simulink model "PMSM_LPVmethods_checked"  (R2023b)
settings: Solver=ode4  StartTime=0.0  StopTime=15  FixedStep=1e-4  RelTol=1e-3
undefined symbols (not defined in the file): Ae1, Ae2, Ae3, Ae4, B, ControlMode_Elec, ControlMode_Mech, Current_Control, J, K1, k1_CST, K2, K3, K4, kd_elec, ki_elec, Km, kp_elec, L, Nr, OmegaStar_Selector, R, sigma1, sigma2, theta0, Vhatinv, Vmax
libraries: simulink x8, slpidlib x2
settings Model: Creator=ghwls  LastModifiedBy=HoLab
settings SolverCC: AlgebraicLoopSolver=TrustRegion
settings DataIOCC: SaveFormat=StructureWithTime  ReturnWorkspaceOutputs=off
settings DebuggingCC: UnconnectedInputMsg=warning  UnconnectedOutputMsg=warning  UnconnectedLineMsg=warning  ArithmeticOperatorsInVariantConditions=warning
settings ModelReferenceCC: EnableRefExpFcnMdlSchedulingChecks=on
settings SFSimCC: CustomCodeUndefinedFunction=UseInterfaceOnly

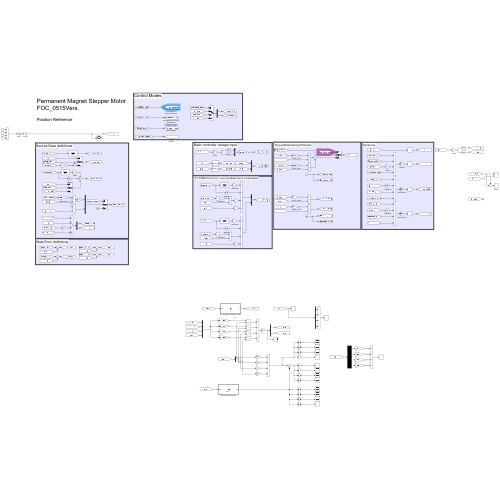
[thumbnail: Simulink's stored preview of the top-level diagram]
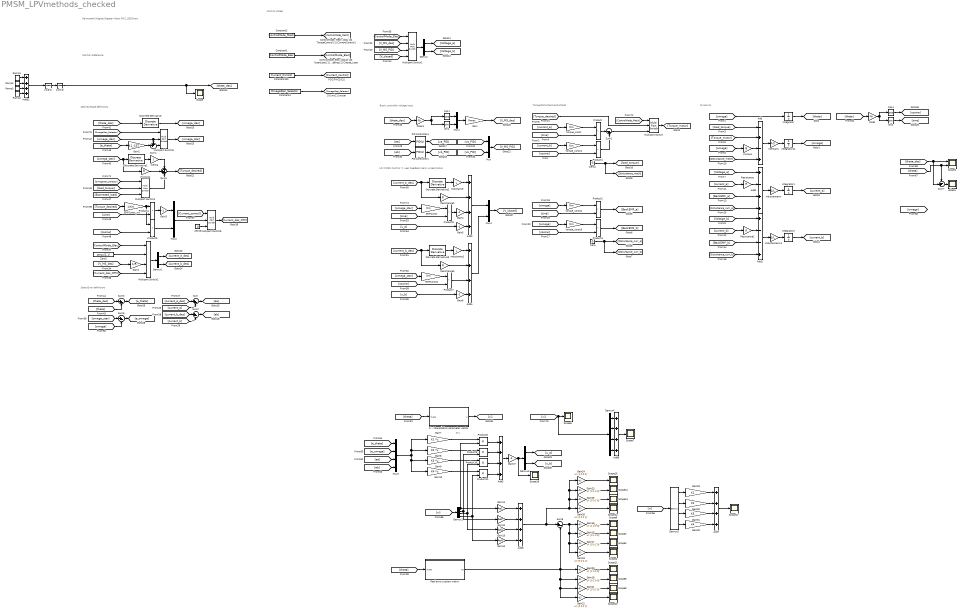
== system PMSM_LPVmethods_checked ==
  note: 2*1
  note: Control Modes
  note: Dynamics
  note: Permanent Magnet Stepper Motor
      | FOC_0515Vers.
  note: Torque/Disturbances/Purterbs
  note: Position Reference
  note: Desired State definitions
  note: Basic controller voltage input
  note: State Error definitions
  note: LPV PMSM Control (Y. Lee) Feedback Semi Liniearization
  Add : Sum  Inputs=-+-+
  Add1 : Sum  Inputs=+-++
  Add2 : Sum  Inputs=+--+
  Add3 : Sum  Inputs=++++
  Add{4..8,32} (6 alike) : Sum  Inputs=4
  Constant1 : Constant  Value=ControlMode_Elec
  Constant100 : Constant  Value=Current_Control
  Constant2 : Constant  Value=ControlMode_Mech
  Constant4 : Constant  Value=OmegaStar_Selector
  Cos1 : Trigonometry  Operator=cos
  Cos4 : Trigonometry  Operator=cos
  Demux : Demux  Outputs=2
  Demux1 : Demux  Outputs=2
  Demux2 : Demux
  Demux3 : Demux  Outputs=2
  Demux4 : Demux
  Demux5 : Demux
  Discrete Derivative{,1..3} (4 alike) : simulink/Discrete/Discrete Derivative  gainval=1.0  ICPrevScaledInput=0.0  OutMin=[]  OutMax=[]  OutDataType=fixdt(1, 16)  OutScaling=2^-10  DoSatur=off
  EMFConst : Gain  Gain=Km
  EMFConst2 : Gain  Gain=Km
  EMFConst_Inv : Gain  Gain=1/Km
  Gain : Gain  Gain=Vmax
  Gain1 : Gain  Gain=1/R
  Gain10 : Gain  Gain=K4  Multiplication=Matrix(K*u) (u vector)
  Gain11 : Gain  Gain=Ae1
  Gain12 : Gain  Gain=Ae2
  Gain13 : Gain  Gain=Ae3
  Gain14 : Gain  Gain=Ae4
  Gain15 : Gain  Gain=[0 1 0 0]'  Multiplication=Matrix(u*K)
  Gain16 : Gain  Gain=[1 0 0 0]'  Multiplication=Matrix(u*K)
  Gain17 : Gain  Gain=[0 0 1 0]'  Multiplication=Matrix(u*K)
  Gain18 : Gain  Gain=[0 0 0 1]'  Multiplication=Matrix(u*K)
  Gain19 : Gain  Gain=[0 1 0 0]'  Multiplication=Matrix(u*K)
  Gain2 : Gain  Gain=k1_CST
  Gain20 : Gain  Gain=[1 0 0 0]'  Multiplication=Matrix(u*K)
  Gain21 : Gain  Gain=[0 0 1 0]'  Multiplication=Matrix(u*K)
  Gain22 : Gain  Gain=[0 0 0 1]'  Multiplication=Matrix(u*K)
  Gain23 : Gain  Gain=[0 1 0 0]'  Multiplication=Matrix(u*K)
  Gain24 : Gain  Gain=[1 0 0 0]'  Multiplication=Matrix(u*K)
  Gain25 : Gain  Gain=[0 0 1 0]'  Multiplication=Matrix(u*K)
  Gain26 : Gain  Gain=[0 0 0 1]'  Multiplication=Matrix(u*K)
  Gain{3..6,27} (5 alike) : Gain  Gain=-1
  Gain28 : Gain  Gain=K4
  Gain29 : Gain  Gain=K1
  Gain30 : Gain  Gain=K2
  Gain31 : Gain  Gain=K3
  Gain7 : Gain  Gain=K1  Multiplication=Matrix(K*u) (u vector)
  Gain8 : Gain  Gain=K2  Multiplication=Matrix(K*u) (u vector)
  Gain9 : Gain  Gain=K3  Multiplication=Matrix(K*u) (u vector)
  Inductance : Gain  Gain=L
  Inductance1 : Gain  Gain=L
  InductanceInv : Gain  Gain=1/L
  InductanceInv1 : Gain  Gain=1/L
  Inertia : Gain  Gain=J
  InertiaInv : Gain  Gain=1/J
  Integrator : Integrator  InitialCondition=theta0
  Integrator1 : Integrator
  Integrator11 : Integrator
  Integrator2 : Integrator
  Multiport Switch{,3..5} (4 alike) : MultiPortSwitch  DataPortOrder=Zero-based contiguous  Inputs=2  zeroidx=on  SaturateOnIntegerOverflow=off  InputSameDT=off
  Multiport Switch1 : MultiPortSwitch  DataPortOrder=Zero-based contiguous  zeroidx=on  SaturateOnIntegerOverflow=off  InputSameDT=off
  Multiport Switch2 : MultiPortSwitch  DataPortOrder=Zero-based contiguous  zeroidx=on  SaturateOnIntegerOverflow=off  InputSameDT=off
  Mux{,1..2,4} (4 alike) : Mux  Inputs=2
  Mux3 : Mux
  PID Controller1 : slpidlib/PID Controller  Controller=PID  Form=Parallel  TimeDomain=Continuous-time  UseExternalTs=off  SampleTime=-1  IntegratorMethod=Forward Euler  FilterMethod=Forward Euler  ControllerParametersSource=internal  P=kp_elec  I=ki_elec  UseKiTs=off  D=kd_elec  N=100  UseFilter=on  TunerSelectOption=Transfer Function Based (PID Tuner App)  ZeroCross=off  InitialConditionSource=internal  InitialConditionForIntegrator=0  InitialConditionForFilter=0  DifferentiatorICPrevScaledInput=0  ExternalReset=none  TrackingMode=off  Kt=1  LimitOutput=off  SatLimitsSource=internal  UpperSaturationLimit=inf  LowerSaturationLimit=-inf  LinearizeAsGain=on  AntiWindupMode=none  Kb=1  LimitIntegrator=off  UpperIntegratorSaturationLimit=inf  LowerIntegratorSaturationLimit=-inf  POutMin=[]  POutMax=[]  IOutMin=[]  IOutMax=[]  DOutMin=[]  DOutMax=[]  NOutMin=[]  NOutMax=[]  SumOutMin=[]  SumOutMax=[]  SaturationOutMin=[]  SaturationOutMax=[]  PParamMin=[]  PParamMax=[]  IParamMin=[]  IParamMax=[]  DParamMin=[]  DParamMax=[]  NParamMin=[]  NParamMax=[]  KbParamMin=[]  KbParamMax=[]  KtParamMin=[]  KtParamMax=[]  KbOutMin=[]  KbOutMax=[]  KtOutMin=[]  KtOutMax=[]  IntegratorOutMin=[]  IntegratorOutMax=[]  FilterOutMin=[]  FilterOutMax=[]  SumI1OutMin=[]  SumI1OutMax=[]  SumI2OutMin=[]  SumI2OutMax=[]  SumI3OutMin=[]  SumI3OutMax=[]  SumI4OutMin=[]  SumI4OutMax=[]  SumDOutMin=[]  SumDOutMax=[]  DifferentiatorOutMin=[]  DifferentiatorOutMax=[]  FilterDiffOutCoefMin=[]  FilterDiffOutCoefMax=[]  ReciprocalOutMin=[]  ReciprocalOutMax=[]  SumDenOutMin=[]  SumDenOutMax=[]  SumNumOutMin=[]  SumNumOutMax=[]  DivideOutMin=[]  DivideOutMax=[]  UdiffTsProdOutMin=[]  UdiffTsProdOutMax=[]  NTsProdOutMin=[]  NTsProdOutMax=[]  UintegralTsProdOutMin=[]  UintegralTsProdOutMax=[]  UngainTsProdOutMin=[]  UngainTsProdOutMax=[]  ClampingZeroOutDataTypeStr=Inherit: Inherit via back propagation  ClampingZeroOutMin=[]  ClampingZeroOutMax=[]  FilterDenConstantOutDataTypeStr=Inherit: Inherit via back propagation  FilterDenConstantOutMin=[]  FilterDenConstantOutMax=[]  PCopyOutDataTypeStr=Inherit: Inherit via back propagation  PCopyOutMin=[]  PCopyOutMax=[]  NCopyOutDataTypeStr=Inherit: Inherit via back propagation  NCopyOutMin=[]  NCopyOutMax=[]  IntegratorContinuousStateAttributes=''  IntegratorStateMustResolveToSignalObject=off  IntegratorRTWStateStorageClass=Auto  FilterContinuousStateAttributes=''  FilterStateMustResolveToSignalObject=off  FilterRTWStateStorageClass=Auto  ParallelPVariant=InternalParameters  IdealPVariant=Disabled  IVariant=InternalParameters  DVariant=InternalParameters  IntegratorVariant=Continuous  SatVariant=Disabled  AWVariant=Passthrough  PCopyVariant=Disabled  TRVariant=Disabled  FdbkBlocksVariant=Forward  IdealPFdbkVariant=Disabled  SatFdbkVariant=Disabled  DerivativeFilterVariant=ContFilter  NVariant=InternalParameters  NCopyVariant=Disabled  FilterICVariant=InternalICsFilter  IntegratorICVariant=InternalICs  ExternalResetVariant=Disabled  TRSumVariant=Passthrough  SumFdbkVariant=Disabled  SumVariant=Sum_PID  TsampFilterVariant=InternalTs  TsampNgainVariant=Passthrough  TsampIntegralVariant=Disabled_SignalSpec  ExternalSaturationOutDataTypeStr=Inherit: Same as second input
  PID Controller4 : slpidlib/PID Controller  Controller=PID  Form=Parallel  TimeDomain=Continuous-time  UseExternalTs=off  SampleTime=-1  IntegratorMethod=Forward Euler  FilterMethod=Forward Euler  ControllerParametersSource=internal  P=kp_elec  I=ki_elec  UseKiTs=off  D=kd_elec  N=100  UseFilter=on  TunerSelectOption=Transfer Function Based (PID Tuner App)  ZeroCross=off  InitialConditionSource=internal  InitialConditionForIntegrator=0  InitialConditionForFilter=0  DifferentiatorICPrevScaledInput=0  ExternalReset=none  TrackingMode=off  Kt=1  LimitOutput=off  SatLimitsSource=internal  UpperSaturationLimit=inf  LowerSaturationLimit=-inf  LinearizeAsGain=on  AntiWindupMode=none  Kb=1  LimitIntegrator=off  UpperIntegratorSaturationLimit=inf  LowerIntegratorSaturationLimit=-inf  POutMin=[]  POutMax=[]  IOutMin=[]  IOutMax=[]  DOutMin=[]  DOutMax=[]  NOutMin=[]  NOutMax=[]  SumOutMin=[]  SumOutMax=[]  SaturationOutMin=[]  SaturationOutMax=[]  PParamMin=[]  PParamMax=[]  IParamMin=[]  IParamMax=[]  DParamMin=[]  DParamMax=[]  NParamMin=[]  NParamMax=[]  KbParamMin=[]  KbParamMax=[]  KtParamMin=[]  KtParamMax=[]  KbOutMin=[]  KbOutMax=[]  KtOutMin=[]  KtOutMax=[]  IntegratorOutMin=[]  IntegratorOutMax=[]  FilterOutMin=[]  FilterOutMax=[]  SumI1OutMin=[]  SumI1OutMax=[]  SumI2OutMin=[]  SumI2OutMax=[]  SumI3OutMin=[]  SumI3OutMax=[]  SumI4OutMin=[]  SumI4OutMax=[]  SumDOutMin=[]  SumDOutMax=[]  DifferentiatorOutMin=[]  DifferentiatorOutMax=[]  FilterDiffOutCoefMin=[]  FilterDiffOutCoefMax=[]  ReciprocalOutMin=[]  ReciprocalOutMax=[]  SumDenOutMin=[]  SumDenOutMax=[]  SumNumOutMin=[]  SumNumOutMax=[]  DivideOutMin=[]  DivideOutMax=[]  UdiffTsProdOutMin=[]  UdiffTsProdOutMax=[]  NTsProdOutMin=[]  NTsProdOutMax=[]  UintegralTsProdOutMin=[]  UintegralTsProdOutMax=[]  UngainTsProdOutMin=[]  UngainTsProdOutMax=[]  ClampingZeroOutDataTypeStr=Inherit: Inherit via back propagation  ClampingZeroOutMin=[]  ClampingZeroOutMax=[]  FilterDenConstantOutDataTypeStr=Inherit: Inherit via back propagation  FilterDenConstantOutMin=[]  FilterDenConstantOutMax=[]  PCopyOutDataTypeStr=Inherit: Inherit via back propagation  PCopyOutMin=[]  PCopyOutMax=[]  NCopyOutDataTypeStr=Inherit: Inherit via back propagation  NCopyOutMin=[]  NCopyOutMax=[]  IntegratorContinuousStateAttributes=''  IntegratorStateMustResolveToSignalObject=off  IntegratorRTWStateStorageClass=Auto  FilterContinuousStateAttributes=''  FilterStateMustResolveToSignalObject=off  FilterRTWStateStorageClass=Auto  ParallelPVariant=InternalParameters  IdealPVariant=Disabled  IVariant=InternalParameters  DVariant=InternalParameters  IntegratorVariant=Continuous  SatVariant=Disabled  AWVariant=Passthrough  PCopyVariant=Disabled  TRVariant=Disabled  FdbkBlocksVariant=Forward  IdealPFdbkVariant=Disabled  SatFdbkVariant=Disabled  DerivativeFilterVariant=ContFilter  NVariant=InternalParameters  NCopyVariant=Disabled  FilterICVariant=InternalICsFilter  IntegratorICVariant=InternalICs  ExternalResetVariant=Disabled  TRSumVariant=Passthrough  SumFdbkVariant=Disabled  SumVariant=Sum_PID  TsampFilterVariant=InternalTs  TsampNgainVariant=Passthrough  TsampIntegralVariant=Disabled_SignalSpec  ExternalSaturationOutDataTypeStr=Inherit: Same as second input
  Poles : Gain  Gain=Nr
  Poles1 : Gain  Gain=Nr
  Product{,1..11} (12 alike) : Product
  Ramp1 : simulink/Sources/Ramp  slope=0.06  start=1  InitialOutput=0
  Ramp2 : simulink/Sources/Ramp  slope=-0.06  start=4  InitialOutput=0
  Ramp3 : simulink/Sources/Ramp  slope=-0.06  start=6  InitialOutput=0
  Ramp4 : simulink/Sources/Ramp  slope=0.06  start=10  InitialOutput=0
  Real error system matrix : MATLAB Function  TreatAsAtomicUnit=on
  Resistance{,1..3} (4 alike) : Gain  Gain=R
  Scope{,2..17} (17 alike) : Scope
  Scope1 : Scope  NumInputPorts=2
  Sin1 : Trigonometry
  Sin4 : Trigonometry
  Sum{,2..3,6,8} (5 alike) : Sum  Inputs=|+-
  Sum1 : Sum  Inputs=|-+
  Sum4 : Sum  Inputs=++|
  Sum5 : Sum  Inputs=+++
  Sum7 : Sum  Inputs=-+|
  Viscous : Gain  Gain=B
  Viscous1 : Gain  Gain=B
  Xi - interpolation parameter vector : MATLAB Function  TreatAsAtomicUnit=on
  Zero : Constant  Value=0  OutDataTypeStr=Inherit: Inherit via back propagation
  Zero1 : Constant  Value=0  OutDataTypeStr=Inherit: Inherit via back propagation
  Zero2 : Constant  Value=zeros(2,1)  OutDataTypeStr=Inherit: Inherit via back propagation
  Zero3 : Constant  Value=0  OutDataTypeStr=Inherit: Inherit via back propagation
  etheta : Scope
  s=5(1) : TransferFcn  Numerator=[5]  Denominator=[1 5]
  s=5(2) : TransferFcn  Numerator=[5]  Denominator=[1 5]
  torque_const{,1..3} (4 alike) : Gain  Gain=Km
  wires:
  [current_a] -> torque_const/1
  InertiaInv/1 -> Integrator11/1
  Integrator11/1 -> [omega]
  Integrator/1 -> [theta]
  Add/1 -> InertiaInv/1
  torque_const/1 -> Product/1
  [omega] -> Integrator/1
  [current_b] -> torque_const1/1
  Sin4/1 -> [sine]
  [theta] -> Poles/1
  Cos4/1 -> [cosine]
  [sine] -> Product/2
  Sum1/1 -> Multiport Switch/3
  Product/1 -> Sum1/1
  Product1/1 -> Sum1/2
  torque_const1/1 -> Product1/1
  [cosine] -> Product1/2
  [load_torque] -> Add/1
  [Torque_motor] -> Add/2
  [Disturbance_mech] -> Add/4
  Viscous/1 -> Add/3
  [omega] -> Viscous/1
  Integrator1/1 -> [current_a]
  Integrator2/1 -> [current_b]
  InductanceInv/1 -> Integrator1/1
  InductanceInv1/1 -> Integrator2/1
  Add1/1 -> InductanceInv/1
  Add2/1 -> InductanceInv1/1
  [Voltage_a] -> Add1/1
  [Voltage_b] -> Add2/1
  Resistance/1 -> Add1/2
  [current_a] -> Resistance/1
  Resistance1/1 -> Add2/2
  [current_b] -> Resistance1/1
  [BackEMF_a] -> Add1/3
  [BackEMF_b] -> Add2/3
  [Disturbance_curr_a] -> Add1/4
  [Disturbance_curr_b] -> Add2/4
  Zero/1 -> [Disturbance_curr_b], [Disturbance_curr_a]
  [cosine] -> Product3/2
  torque_const3/1 -> Product3/1
  [sine] -> Product2/2
  [omega] -> torque_const3/1
  torque_const2/1 -> Product2/1
  [omega] -> torque_const2/1
  Product2/1 -> [BackEMF_a]
  Product3/1 -> [BackEMF_b]
  Zero1/1 -> [load_torque], [Disturbance_mech]
  Multiport Switch/1 -> [Torque_motor]
  [Torque_desired] -> Multiport Switch/2
  Multiport Switch1/1 -> Demux/1
  Demux/1 -> [Voltage_a]
  Demux/2 -> [Voltage_b]
  [V_MS_des] -> Multiport Switch1/2
  [V_MS_PID] -> Multiport Switch1/3
  [V_closed] -> Multiport Switch1/4
  [current_a_des] -> Sum/1
  [current_a] -> Sum/2
  [current_b_des] -> Sum2/1
  [current_b] -> Sum2/2
  Sum/1 -> [ea]
  Sum2/1 -> [eb]
  [ea] -> PID Controller4/1
  [eb] -> PID Controller1/1
  PID Controller4/1 -> [va_PID]
  PID Controller1/1 -> [vb_PID]
  [vb_PID] -> Mux/2
  [va_PID] -> Mux/1
  Mux/1 -> [V_MS_PID]
  Poles/1 -> Sin4/1, Cos4/1
  Poles1/1 -> Cos1/1, Sin1/1
  Cos1/1 -> Mux1/1
  [theta_des] -> Poles1/1
  Sin1/1 -> Mux1/2
  Mux1/1 -> Gain/1
  Gain/1 -> [V_MS_des]
  [V_MS_des] -> Gain1/1
  Demux1/1 -> [current_a_des]
  Demux1/2 -> [current_b_des]
  Multiport Switch2/1 -> Demux1/1
  [ControlMode_Elec] -> Multiport Switch2/1
  [ControlMode_Elec] -> Multiport Switch1/1
  Constant1/1 -> [ControlMode_Elec]
  [ControlMode_Mech] -> Multiport Switch/1
  Constant2/1 -> [ControlMode_Mech]
  Gain1/1 -> Multiport Switch2/3
  Zero2/1 -> Multiport Switch2/2
  [Current_des_NTM] -> Multiport Switch2/4
  [theta_des] -> Discrete Derivative/1
  Discrete Derivative/1 -> [omega_des]
  Multiport Switch3/1 -> [omega_star]
  [omega_des] -> Multiport Switch3/2, Sum4/1
  [theta_des] -> Sum3/1
  [theta] -> Sum3/2
  Sum3/1 -> [e_theta]
  [e_theta] -> Gain2/1
  Gain2/1 -> Sum4/2
  Sum4/1 -> Multiport Switch3/3
  [OmegaStar_Selector] -> Multiport Switch3/1
  [omega_star] -> Viscous1/1, Discrete Derivative1/1
  Discrete Derivative1/1 -> Inertia/1
  [load_torque] -> Multiport Switch4/2
  [Estimated_load] -> Multiport Switch4/3
  [OmegaStar_Selector] -> Multiport Switch4/1
  Viscous1/1 -> Sum5/2
  Inertia/1 -> Sum5/1
  Multiport Switch4/1 -> Sum5/3
  [Torque_desired] -> EMFConst_Inv/1
  EMFConst_Inv/1 -> Product5/1, Product4/1
  [sine] -> Product4/2
  [cosine] -> Product5/2
  Product4/1 -> Gain3/1
  Gain3/1 -> Mux2/1
  Product5/1 -> Mux2/2
  Multiport Switch5/1 -> [Current_des_NTM]
  Mux2/1 -> Multiport Switch5/2
  Zero3/1 -> Multiport Switch5/3
  Mux4/1 -> [V_closed]
  [current_a_des] -> Resistance2/1, Discrete Derivative2/1
  Discrete Derivative2/1 -> Inductance/1
  Gain4/1 -> Add3/3
  Product6/1 -> Gain4/1
  [sine] -> Product6/2
  EMFConst/1 -> Product6/1
  [omega_star] -> EMFConst/1
  Inductance/1 -> Add3/1
  Resistance2/1 -> Add3/2
  Add3/1 -> Mux4/1
  Resistance3/1 -> Add4/2
  Inductance1/1 -> Add4/1
  EMFConst2/1 -> Product7/1
  [cosine] -> Product7/2
  Discrete Derivative3/1 -> Inductance1/1
  [current_b_des] -> Resistance3/1, Discrete Derivative3/1
  [omega_star] -> EMFConst2/1
  Add4/1 -> Mux4/2
  Gain5/1 -> Add3/4
  Gain6/1 -> Add4/4
  Constant100/1 -> [Current_control]
  [Current_control] -> Multiport Switch5/1
  [omega_star] -> Sum6/1
  [omega] -> Sum6/2
  Sum6/1 -> [e_omega]
  [theta] -> Xi - interpolation parameter vector/1(theta)
  Xi - interpolation parameter vector/1(xi) -> [xi]
  [e_theta] -> Mux3/1
  [e_omega] -> Mux3/2
  [ea] -> Mux3/3
  [eb] -> Mux3/4
  Mux3/1 -> Gain10/1, Gain9/1, Gain8/1, Gain7/1
  [xi] -> Demux2/1
  Gain7/1 -> Product8/1
  Gain8/1 -> Product9/1
  Gain9/1 -> Product10/1
  Gain10/1 -> Product11/1
  Demux2/1 -> Product8/2, Gain11/1
  Demux2/2 -> Product9/2, Gain12/1
  Demux2/3 -> Product10/2, Gain13/1
  Demux2/4 -> Product11/2, Gain14/1
  Product8/1 -> Add5/1
  Product9/1 -> Add5/2
  Product10/1 -> Add5/3
  Product11/1 -> Add5/4
  Add5/1 -> Gain27/1
  Demux3/1 -> [u_a]
  Demux3/2 -> [u_b]
  [theta_des] -> Sum7/2, Scope1/1
  [theta] -> Scope1/2, Sum7/1
  Constant4/1 -> [OmegaStar_Selector]
  Gain11/1 -> Add6/1
  Gain12/1 -> Add6/2
  Gain13/1 -> Add6/3
  Gain14/1 -> Add6/4
  [theta] -> Real error system matrix/1(theta)
  Real error system matrix/1(Ae) -> Gain22/1, Gain21/1, Gain19/1, Gain20/1, Sum8/2
  Sum8/1 -> Gain18/1, Gain17/1, Gain15/1, Gain16/1
  Gain16/1 -> Scope6/1
  Gain15/1 -> Scope2/1
  Gain17/1 -> Scope3/1
  Gain18/1 -> Scope4/1
  [xi] -> Demux4/1, Scope5/1
  Demux4/1 -> Add8/1
  Demux4/2 -> Add8/2
  Demux4/3 -> Add8/3
  Demux4/4 -> Add8/4
  Add8/1 -> Scope7/1
  Gain22/1 -> Scope10/1
  Gain21/1 -> Scope9/1
  Gain19/1 -> Scope8/1
  Gain20/1 -> Scope11/1
  Gain26/1 -> Scope14/1
  Gain25/1 -> Scope13/1
  Gain23/1 -> Scope12/1
  Gain24/1 -> Scope15/1
  Add6/1 -> Gain24/1, Gain23/1, Gain25/1, Gain26/1, Sum8/1
  Product7/1 -> Add4/3
  Sum5/1 -> [Torque_desired]
  Gain27/1 -> Scope16/1, Demux3/1
  Sum7/1 -> etheta/1
  Add32/1 -> s=5(1)/1
  Ramp3/1 -> Add32/3
  Ramp2/1 -> Add32/2
  s=5(1)/1 -> s=5(2)/1
  Ramp1/1 -> Add32/1
  Ramp4/1 -> Add32/4
  s=5(2)/1 -> Scope/1, [theta_des]
  [u_a] -> Gain5/1
  [u_b] -> Gain6/1
  [xi] -> Demux5/1
  Demux5/1 -> Gain29/1
  Demux5/2 -> Gain30/1
  Demux5/3 -> Gain31/1
  Demux5/4 -> Gain28/1
  Gain29/1 -> Add7/1
  Gain30/1 -> Add7/2
  Gain31/1 -> Add7/3
  Gain28/1 -> Add7/4
  Add7/1 -> Scope17/1

== matlab function PMSM_LPVmethods_checked/Real error system matrix ==
  data: theta input; B parameter; Km parameter; J parameter; Nr parameter; R parameter; Ae output; L parameter
function Ae = fcn(theta,B,Km,J,Nr,R,L)

Ae = [0 1 0 0;0 -B/J -Km/J*sin(Nr*theta) Km/J*cos(Nr*theta); 0 Km/L*sin(Nr*theta) -R/L 0;0 -Km/L*cos(Nr*theta) 0 -R/L];

== matlab function PMSM_LPVmethods_checked/Xi - interpolation parameter vector ==
  data: theta input; Vhatinv parameter; sigma1 parameter; sigma2 parameter; xi output; Km parameter; Nr parameter
function xi = fcn(theta, Vhatinv, sigma1, sigma2, Km, Nr)
eta1 = Km*sin(Nr*theta);
eta2 = Km*cos(Nr*theta);
etahat = [[eta1 eta2] sigma1 sigma2]';
xi = Vhatinv*etahat;
